simulink model "rsx_sat_sim"  (R2025a)
settings: Solver=VariableStepAuto  StartTime=0.0  StopTime=20  RelTol=1e-3
undefined symbols (not defined in the file or in its folder): K, K_c
libraries: simulink_extras x2
settings Model: Creator=layer  LastModifiedBy=layer

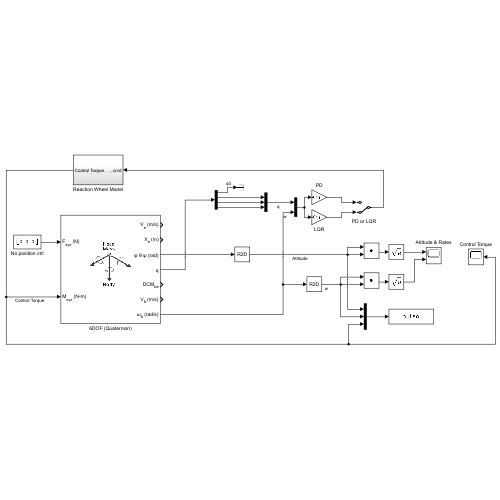
[thumbnail: Simulink's stored preview of the top-level diagram]
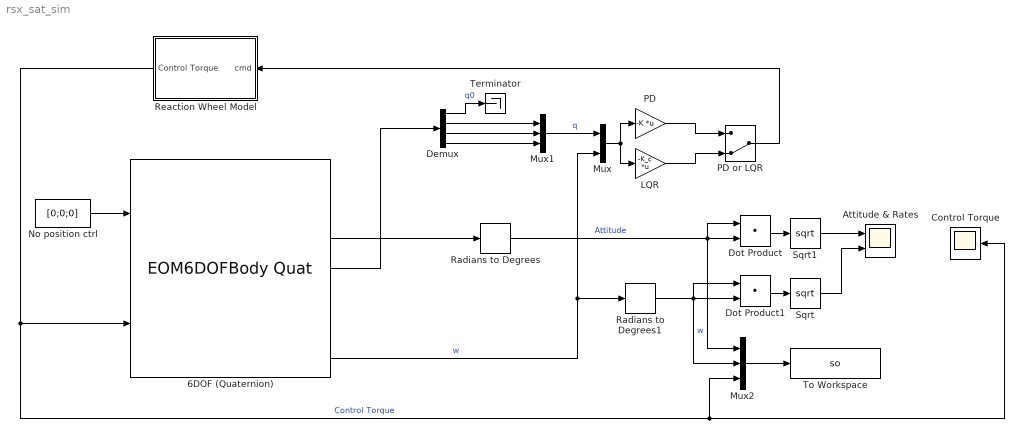
== system rsx_sat_sim ==
  6DOF (Quaternion) : EOM6DOFBodyQuat  eul_0=[pi/3 pi/3 pi/3]  pm_0=[0.0 0.0 0.0]  inertia=J
  Attitude & Rates : Scope  NumInputPorts=2
      settings: ActiveDisplayYMinimum=-79.961862192550882  ActiveDisplayYMaximum=107.5739063763623
  Control Torque : Scope
      settings: ActiveDisplayYMinimum=-0.0062499999999999995  ActiveDisplayYMaximum=0.0062499999999999995
  Demux : Demux
  Dot Product : DotProduct  OutDataTypeStr=Inherit: Inherit via internal rule
  Dot Product1 : DotProduct  OutDataTypeStr=Inherit: Inherit via internal rule
  LQR : Gain  Gain=-K_c  Multiplication=Matrix(K*u)
  Mux : Mux  Inputs=2
  Mux1 : Mux  Inputs=3
  Mux2 : Mux  Inputs=3
  No position ctrl : Constant  Value=[0;0;0]  SampleTime=0.1
  PD : Gain  Gain=-K  Multiplication=Matrix(K*u)
  PD or LQR : ManualSwitch  CurrentSetting=0
  Radians to Degrees : simulink_extras/Transformations/Radians to Degrees
  Radians to Degrees1 : simulink_extras/Transformations/Radians to Degrees
  Reaction Wheel Model : Subsystem
  Sqrt : Sqrt
  Sqrt1 : Sqrt
  Terminator : Terminator
  To Workspace : ToWorkspace  VariableName=so  SaveFormat=Structure With Time  SampleTime=-1
      settings: Decimation=2
  wires:
  Demux/1 -> Terminator/1  "q0"
  Demux/2 -> Mux1/1
  Demux/3 -> Mux1/2
  Demux/4 -> Mux1/3
  No position ctrl/1 -> 6DOF (Quaternion)/1
  6DOF (Quaternion)/7 -> Mux/2, Radians to Degrees1/1  "w"
  Mux1/1 -> Mux/1  "q"
  6DOF (Quaternion)/4 -> Demux/1
  Mux/1 -> LQR/1, PD/1
  6DOF (Quaternion)/3 -> Radians to Degrees/1
  Radians to Degrees/1 -> Mux2/1, Dot Product/2, Dot Product/1  "Attitude"
  PD/1 -> PD or LQR/1
  LQR/1 -> PD or LQR/2
  Radians to Degrees1/1 -> Dot Product1/1, Dot Product1/2, Mux2/2  "w"
  Mux2/1 -> To Workspace/1
  Sqrt1/1 -> Attitude & Rates/1
  Sqrt/1 -> Attitude & Rates/2
  Dot Product1/1 -> Sqrt/1
  Dot Product/1 -> Sqrt1/1
  Reaction Wheel Model/1(Control Torque) -> Control Torque/1, Mux2/3, 6DOF (Quaternion)/2  "Control Torque"
  PD or LQR/1 -> Reaction Wheel Model/1(cmd)

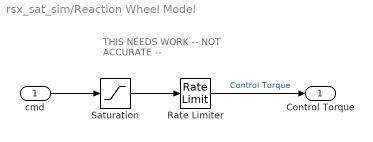
== system rsx_sat_sim/Reaction Wheel Model ==
  note: THIS NEEDS WORK
      | -- NOT ACCURATE --
  cmd : Inport
  Rate Limiter : RateLimiter  RisingSlewLimit=0.1  FallingSlewLimit=-0.1  SampleTimeMode=inherited
  Saturation : Saturate  UpperLimit=0.005  LowerLimit=-0.005
  Control Torque : Outport
  wires:
  Saturation/1 -> Rate Limiter/1
  cmd/1 -> Saturation/1
  Rate Limiter/1 -> Control Torque/1  "Control Torque"
